simulink model "helicopter_sim"  (R2024b)
settings: Solver=ode4  StartTime=0.0  StopTime=30  FixedStep=ST  RelTol=1e-3
StopFcn:
  | % main rotor flapping restraint
  | if over_flap
  |     warning('MyModel:flapping', '<strong> main rotor blade flapping exceeded limits </strong>');
  | end
  | % tail rotor flapping restraint
  | if over_flap_tr
  |     warning('MyModel:flapping_tr', '<strong> tail rotor blade flapping exceeded limits </strong>');
  | end
  | % main rotor load limit
  | if load_mr
  |     warning('MyModel:load_mr', '<strong> main rotor load limit reached </strong>');
  | end
  | % main rotor power limit
  | if power_mr
  |     warning('MyModel:power_mr', '<strong> transmission maximum power rating reached </strong>');
  | end
  | % main rotor blade stall
  | if stall_mr
  |     warning('MyModel:blade_stall', '<strong> main rotor blade stall </strong>');
  | end
  | clear over_flap over_flap_tr load_mr power_mr stall_mr
values from neighbouring files (symbols this model uses):
  a_0 = [ 0 0 0 ]'*pi/180    [parameters.m]    (also in trim.m = [ flap_ss(1) flap_ss(2) flap_ss(3) ]')
  a_hs = 6    [parameters.m]
  a_vs = 6    [parameters.m]
  AKBETA = 0    [parameters.m]
  AKONE = 0    [parameters.m]
  AKONETR = tan(30*(pi/180))    [parameters.m]
  alpha_stall = 15    [parameters.m]
  AOP = 0    [parameters.m]
  AOPTR = 0    [parameters.m]
  AR_hs = 4.5    [parameters.m]
  AR_vs = 1.8    [parameters.m]
  ASLOPE = 6    [parameters.m]
  ASLOPETR = 6    [parameters.m]
  BLADES = 4    [parameters.m]
  BLADESTR = 3    [parameters.m]
  BLCG = 0    [parameters.m]
  BLHS = 0    [parameters.m]
  BLMR = 0    [parameters.m]
  BLRPF = 0    [parameters.m]
  BLTR = -1.8*Ft_m    (= -0.54864)    [parameters.m]
  BLVS = 0    [parameters.m]
  CD_f = [1.774 0.2043 7]    [parameters.m]
  CD_mr = [0.0107 -0.151 1.72]    [parameters.m]
  CD_tr = [ 0.0107 -0.151 1.72 ]    [parameters.m]
  chi_mr = 1    [parameters.m]
  chi_tr = 1    [parameters.m]
  CHORD = 2*Ft_m    (= 0.6096)    [parameters.m]
  CHORDTR = 1*Ft_m    (= 0.3048)    [parameters.m]
  CL_f = [-0.4279 10.33]    [parameters.m]
  CL_max_hs = 1.2    [parameters.m]
  CL_max_vs = 1.2    [parameters.m]
  CLL_f = [0.0696 6.336]    [parameters.m]
  CM_f = [-4.4961 49.522]    [parameters.m]
  CN_f = [0.0396 -21.699]    [parameters.m]
  CY_f = [-0.0359 -16.987]    [parameters.m]
  D = zeros(9,4)    [linearization.m]
  dyn_viscosity = 17.89e-6    (= 1.789e-05)    [parameters.m]
  e_hs = 0.8    [parameters.m]
  e_vs = 0.8    [parameters.m]
  EPSLN = 0.05    [parameters.m]
  euler0 = [ 0 0 0 ]'*pi/180    [parameters.m]    (also in trim.m = [ euler_trim(1)*abs(max_att) euler_trim(2)*abs(max_att) eule)
  fc = [  100*Kn_mps ... (first row only)    [parameters.m]
  GAMMA = 8.1    [parameters.m]
  GAMMATR = 4    [parameters.m]
  href = 0    [parameters.m]
  i_hs = -3*(pi/180)+a0_hs    (= -0.0523598775598)    [parameters.m]
  i_s = 0    [parameters.m]
  i_vs = 0*(pi/180)+a0_vs    (= -0.0872664625997)    [parameters.m]
  Jbeta = 1/3*m_blade*ROTOR^3*(1-EPSLN)^3    (= 3891.86391298)    [parameters.m]
  k_ind = 1    [parameters.m]
  k_ind_tr = 1    [parameters.m]
  kv_tr = 0.8    [parameters.m]
  Lambda_hs = 13*(pi/180)    (= 0.226892802759)    [parameters.m]
  Lambda_vs = 27*(pi/180)    (= 0.471238898038)    [parameters.m]
  lat_cyc_range = [ -15 15 ]    [parameters.m]
  latref = 39.24744998520548    (= 39.2474499852)    [parameters.m]
  lon_cyc_range = [ -15 15 ]    [parameters.m]
  lonref = 9.050782438199448    (= 9.0507824382)    [parameters.m]
  m = 20000*Lb_Kg    (= 9071.84)    [parameters.m]
  m_blade = 0.372*Slug_Kg/Ft_m    (= 17.8114564173)    [parameters.m]
  max_flap_mr = 20*pi/180    (= 0.349065850399)    [parameters.m]
  max_flap_tr = 20*pi/180    (= 0.349065850399)    [parameters.m]
  max_load = 3*m*9.81    (= 266984.2512)    [parameters.m]
  mode = 0    [linearization.m]    (also in parameters.m; trim.m)
  mr_coll_range = [   0 25 ]    [parameters.m]
  OMEGA = 206.9*(pi/30)    (= 21.6665173343)    [parameters.m]
  omega0 = [ 0 0 0 ]'    [parameters.m]
  OMEGATR = 954.93*(pi/30)    (= 100.000035756)    [parameters.m]
  pilot_trim = [ x(1); x(2); x(3); x(4) ]    [trim.m]
  rated_power = 4170*hp_W    (= 3109569)    [parameters.m]
  ROTOR = 30*Ft_m    (= 9.144)    [parameters.m]
  ROTORTR = 6.5*Ft_m    (= 1.9812)    [parameters.m]
  S_hs = 18*(Ft_m^2)    (= 1.67225472)    [parameters.m]
  S_vs = 33*(Ft_m^2)    (= 3.06580032)    [parameters.m]
  ST = 0.001    [parameters.m]
  STACG = 24.4*Ft_m    (= 7.43712)    [parameters.m]
  STAHS = 57.4*Ft_m    (= 17.49552)    [parameters.m]
  STAMR = 23.9*Ft_m    (= 7.28472)    [parameters.m]
  STARPF = 23.9*Ft_m    (= 7.28472)    [parameters.m]
  STATR = 61.4*Ft_m    (= 18.71472)    [parameters.m]
  STAVS = 59.4*Ft_m    (= 18.10512)    [parameters.m]
  THETT = -10*(pi/180)    (= -0.174532925199)    [parameters.m]
  THETTTR = -5*(pi/180)    (= -0.0872664625997)    [parameters.m]
  tr_coll_range = [   0 20 ]    [parameters.m]
  Ttrb = [ 1 0 0; 0 0 1; 0 -1 0]    [parameters.m]
  V0 = eul2rotm(euler0','XYZ')'*[ fc(1) fc(2) fc(3) ]'    [parameters.m]    (also in trim.m)
  wind_rate = [ 0 0 0 ]'    [parameters.m]
  wind_velocity_e = [ 0 0 0 ]'    [parameters.m]
  WLCG = 9.2*Ft_m    (= 2.80416)    [parameters.m]
  WLHS = 7.7*Ft_m    (= 2.34696)    [parameters.m]
  WLMR = 16.7*Ft_m    (= 5.09016)    [parameters.m]
  WLRPF = 12.2*Ft_m    (= 3.71856)    [parameters.m]
  WLTR = 15.2*Ft_m    (= 4.63296)    [parameters.m]
  WLVS = 12.2*Ft_m    (= 3.71856)    [parameters.m]
  Xe_0 = [ 16404 0 -1000 ]'*Ft_m    [parameters.m]
undefined symbols (not defined in the file or in its folder): Earth, rad, s, WGS84
libraries: simulink x4, aerolibanimutils x2, aerolibsim3d x2, sim3dlib x1, aerolibconvert2 x1, shared6dof x1, aerolibtransform2 x1, aerolibatmos2 x1
(part 2 of 3)

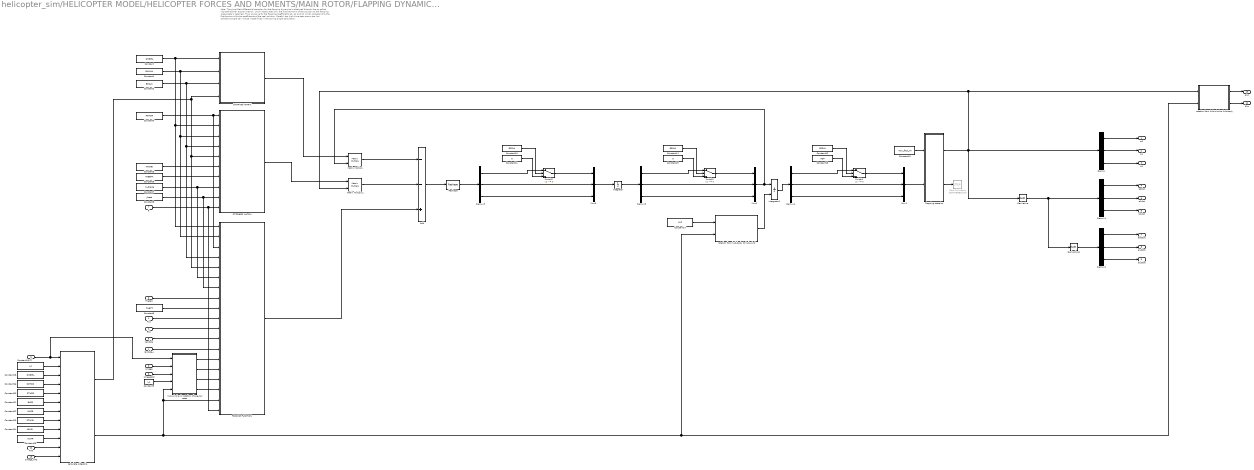
== system helicopter_sim/HELICOPTER MODEL/HELICOPTER FORCES AND MOMENTS/MAIN ROTOR/FLAPPING DYNAMICS (TIP-PATH-PLANE APPROX) ==
  note: Note:
      | The simplified differential equation for the flapping dynamics is obtained through the so called "tip-path-plane" approximation, which means that only the first harmonic of the solution to the flapping angle beta is retained. Thus we solve for the flapping coefficients a0, a1 and b1 which correspond to the first harmonic Fourier coefficients of the real solution.
      | Careful: too high time step size or too low collective angle can induce instabilities in the coning angle calculation.
  A1s : Inport
  B1s : Inport  Port=2
  Theta0 : Inport  Port=3
  lambda_i : Inport  Port=4
  lambda : Inport  Port=5
  chi : Inport  Port=6
  g : Inport  Port=7
  omegadot : Inport  Port=8
  omega : Inport  Port=9
  omega_TAS : Inport  Port=10
  TAS : Inport  Port=11
  Add : Sum  Inputs=--+
  Constant : Constant  Value=OMEGA
  Constant1 : Constant  Value=GAMMA
  Constant{2,10,12,14} (4 alike) : Constant  Value=EPSLN
  Constant11 : Constant  Value=0
  Constant13 : Constant  Value=AOP
  Constant15 : Constant  Value=0
  Constant16 : Constant  Value=max_flap_mr
  Constant17 : Constant  Value=a_0
  Constant18 : Constant  Value=OMEGA
  Constant19 : Constant  Value=i_s
  Constant20 : Constant  Value=STACG
  Constant21 : Constant  Value=BLCG
  Constant22 : Constant  Value=WLCG
  Constant23 : Constant  Value=STAMR
  Constant24 : Constant  Value=BLMR
  Constant25 : Constant  Value=WLMR
  Constant26 : Constant  Value=ROTOR
  Constant3 : Constant  Value=AKONE
  Constant4 : Constant  Value=ROTOR
  Constant5 : Constant  Value=THETT
  Constant6 : Constant  Value=AKBETA
  Constant7 : Constant  Value=m_blade
  Constant8 : Constant  Value=Jbeta
  Constant9 : Constant  Value=i_s
  DAMPING MATRIX : MATLAB Function  TreatAsAtomicUnit=on
  Demux{,1..5} (6 alike) : Demux  Outputs=3
  Derivative : Derivative
  Derivative1 : Derivative
  FORCING FUNCTION : MATLAB Function  TreatAsAtomicUnit=on
  Integrator : Integrator  InitialCondition=[0 0 0]'
  Integrator1 : Integrator  InitialConditionSource=external  InitialCondition=a_0
  Matrix Multiply : Product  Multiplication=Matrix(*)
  Matrix Multiply1 : Product  Multiplication=Matrix(*)
  Mux1 : Mux  Inputs=3
  Mux2 : Mux  Inputs=3
  Mux3 : Mux  Inputs=3
  Reshape : Reshape  OutputDimensionality=Column vector (2-D)
  STIFFNESS MATRIX : MATLAB Function  TreatAsAtomicUnit=on
  Stop Simulation : Stop  Commented=on
  Switch1 : Switch  Criteria=u2 ~= 0  SaturateOnIntegerOverflow=off  InputSameDT=off
  Switch2 : Switch  Criteria=u2 ~= 0  SaturateOnIntegerOverflow=off  InputSameDT=off
  Switch3 : Switch  Criteria=u2 ~= 0  SaturateOnIntegerOverflow=off  InputSameDT=off
  calculate sidesplip : MATLAB Function  TreatAsAtomicUnit=on
  flapping restraint : MATLAB Function  TreatAsAtomicUnit=on
  hub-wind axis rotation of angular rates : MATLAB Function  TreatAsAtomicUnit=on
  rotation from hub-body to hub-wind : MATLAB Function  TreatAsAtomicUnit=on
  rotation from hub-wind to hub-body : MATLAB Function  TreatAsAtomicUnit=on
  a0 : Outport
  a1 : Outport  Port=2
  b1 : Outport  Port=3
  a0dot : Outport  Port=4
  a1dot : Outport  Port=5
  b1dot : Outport  Port=6
  a0ddot : Outport  Port=7
  a1ddot : Outport  Port=8
  b1ddot : Outport  Port=9
  a1s : Outport  Port=10
  b1s : Outport  Port=11
  wires:
  Theta0/1 -> FORCING FUNCTION/8(Theta0)
  Constant2/1 -> DAMPING MATRIX/3(EPSLN), FORCING FUNCTION/4(EPSLN), STIFFNESS MATRIX/4(EPSLN)
  Constant1/1 -> DAMPING MATRIX/2(GAMMA), FORCING FUNCTION/2(GAMMA), STIFFNESS MATRIX/3(GAMMA)
  DAMPING MATRIX/1(D) -> Matrix Multiply/1
  Constant/1 -> FORCING FUNCTION/1(OMEGA), STIFFNESS MATRIX/2(OMEGA), DAMPING MATRIX/1(OMEGA)
  A1s/1 -> FORCING FUNCTION/10(A1s)
  FORCING FUNCTION/1(f) -> Add/3
  STIFFNESS MATRIX/1(K) -> Matrix Multiply1/1
  Constant5/1 -> FORCING FUNCTION/9(THETT)
  Matrix Multiply1/1 -> Add/2
  Demux/2 -> a1/1
  Matrix Multiply/1 -> Add/1
  Demux/1 -> a0/1
  Constant3/1 -> STIFFNESS MATRIX/6(AKONE)
  Demux/3 -> b1/1
  Add/1 -> Reshape/1
  B1s/1 -> FORCING FUNCTION/11(B1s)
  lambda/1 -> FORCING FUNCTION/12(lambda)
  Demux1/3 -> b1dot/1
  Demux1/1 -> a0dot/1
  Demux1/2 -> a1dot/1
  Demux2/2 -> a1ddot/1
  Demux2/1 -> a0ddot/1
  Demux2/3 -> b1ddot/1
  Constant6/1 -> STIFFNESS MATRIX/7(AKBETA)
  Constant7/1 -> STIFFNESS MATRIX/8(m_blade), FORCING FUNCTION/6(m_blade)
  Constant8/1 -> STIFFNESS MATRIX/9(Jbeta), FORCING FUNCTION/7(Jbeta)
  Constant4/1 -> STIFFNESS MATRIX/1(ROTOR), FORCING FUNCTION/3(ROTOR)
  rotation from hub-wind to hub-body/1(a1s) -> a1s/1
  rotation from hub-wind to hub-body/2(b1s) -> b1s/1
  omegadot/1 -> hub-wind axis rotation of angular rates/3(omegadot)
  hub-wind axis rotation of angular rates/1(pW) -> FORCING FUNCTION/14(pW)
  hub-wind axis rotation of angular rates/2(qW) -> FORCING FUNCTION/15(qW)
  hub-wind axis rotation of angular rates/3(pWdot) -> FORCING FUNCTION/16(pWdot)
  hub-wind axis rotation of angular rates/4(qWdot) -> FORCING FUNCTION/17(qWdot)
  omega/1 -> hub-wind axis rotation of angular rates/2(omega)
  Constant9/1 -> hub-wind axis rotation of angular rates/4(i_s)
  calculate sidesplip/1(Mu) -> DAMPING MATRIX/4(Mu), FORCING FUNCTION/5(Mu), STIFFNESS MATRIX/5(Mu)
  g/1 -> STIFFNESS MATRIX/10(g), FORCING FUNCTION/19(g)
  Constant15/1 -> Switch2/3
  Constant14/1 -> Switch2/2
  Demux5/3 -> Mux2/3
  Demux5/2 -> Mux2/2
  Demux5/1 -> Switch2/1
  Switch2/1 -> Mux2/1
  Integrator/1 -> Demux5/1  "adot"
  Mux2/1 -> Matrix Multiply/2, Integrator1/1
  Demux4/1 -> Switch1/1
  Constant13/1 -> Switch1/3
  Constant12/1 -> Switch1/2
  Integrator1/1 -> Demux4/1  "a"
  flapping restraint/1(a) -> Derivative/1, Demux/1, Matrix Multiply1/2, rotation from hub-wind to hub-body/1(a)
  Switch3/1 -> Mux3/1
  Demux3/2 -> Mux3/2
  Demux3/3 -> Mux3/3
  Constant11/1 -> Switch3/3
  Demux3/1 -> Switch3/1
  Constant10/1 -> Switch3/2
  Reshape/1 -> Demux3/1  "addot"
  Mux3/1 -> Integrator/1
  Derivative/1 -> Demux1/1, Derivative1/1
  Derivative1/1 -> Demux2/1
  lambda_i/1 -> FORCING FUNCTION/13(lambda_i)
  Switch1/1 -> Mux1/1
  Demux4/2 -> Mux1/2
  Demux4/3 -> Mux1/3
  Mux1/1 -> flapping restraint/2("a ")
  Constant16/1 -> flapping restraint/1(max_flap)
  flapping restraint/2(stop) -> Stop Simulation/1
  rotation from hub-body to hub-wind/1(a_w) -> Integrator1/2
  Constant17/1 -> rotation from hub-body to hub-wind/1(a_b)
  chi/1 -> hub-wind axis rotation of angular rates/1(chi), calculate sidesplip/1(chi)
  Constant19/1 -> calculate sidesplip/2(i_s)
  Constant20/1 -> calculate sidesplip/5(STACG)
  Constant21/1 -> calculate sidesplip/6(BLCG)
  Constant22/1 -> calculate sidesplip/7(WLCG)
  Constant23/1 -> calculate sidesplip/8(STAH)
  Constant24/1 -> calculate sidesplip/9(BLH)
  Constant25/1 -> calculate sidesplip/10(WLH)
  TAS/1 -> calculate sidesplip/11(TAS)
  Constant18/1 -> calculate sidesplip/3(OMEGA)
  Constant26/1 -> calculate sidesplip/4(ROTOR)
  omega_TAS/1 -> calculate sidesplip/12(omega_TAS)
  calculate sidesplip/2(beta_w) -> FORCING FUNCTION/18(beta_w), hub-wind axis rotation of angular rates/5(beta_w), rotation from hub-body to hub-wind/2(beta_w), rotation from hub-wind to hub-body/2(beta_w)

== system helicopter_sim/HELICOPTER MODEL/HELICOPTER FORCES AND MOMENTS/MAIN ROTOR/Stop simulation if retreating blade stalls  ==
  alpha_loc : Inport
  Compare To Constant : simulink/Logic and Bit Operations/Compare To Constant  relop=>  const=alpha_stall  OutDataTypeStr=boolean
  Display : Display
  MATLAB Function : MATLAB Function  TreatAsAtomicUnit=on
  MATLAB Function1 : MATLAB Function  TreatAsAtomicUnit=on
  Stop Simulation : Stop  Commented=on
  wires:
  Compare To Constant/1 -> MATLAB Function/1(u), Stop Simulation/1
  alpha_loc/1 -> MATLAB Function1/1(alpha_loc)
  MATLAB Function1/1(alpha_max) -> Display/1, Compare To Constant/1

== system helicopter_sim/HELICOPTER MODEL/HELICOPTER FORCES AND MOMENTS/MAIN ROTOR/Stop simulation if main rotor hub load limit is exceeded ==
  T : Inport
  Compare To Constant : simulink/Logic and Bit Operations/Compare To Constant  relop=>  const=max_load  OutDataTypeStr=boolean
  MATLAB Function : MATLAB Function  TreatAsAtomicUnit=on
  Scope : Scope
  Stop Simulation : Stop  Commented=on
  wires:
  Compare To Constant/1 -> MATLAB Function/1(u), Stop Simulation/1
  T/1 -> Scope/1, Compare To Constant/1

== system helicopter_sim/HELICOPTER MODEL/HELICOPTER FORCES AND MOMENTS/MAIN ROTOR/Stop simulation if maximum transmission power rating is exceeded ==
  Q : Inport
  Compare To Constant : simulink/Logic and Bit Operations/Compare To Constant  relop=>  const=rated_power  OutDataTypeStr=boolean
  Constant : Constant  Value=OMEGA
  MATLAB Function : MATLAB Function  TreatAsAtomicUnit=on
  Product : Product
  Scope : Scope
  Stop Simulation : Stop  Commented=on
  wires:
  Compare To Constant/1 -> MATLAB Function/1(u), Stop Simulation/1
  Q/1 -> Product/1
  Constant/1 -> Product/2
  Product/1 -> Compare To Constant/1, Scope/1

== matlab function helicopter_sim/HELICOPTER MODEL/HELICOPTER FORCES AND MOMENTS/STABILIZERS /VERTICAL STABILIZER AERODYNAMIC FORCES AND MOMENTS ==
  data: lambda_i_tr input; TAS input; omega_TAS input; rho input; STAVS input; F_vs output; BLVS input; WLVS input; STACG input; BLCG input; WLCG input; OMEGATR input; ROTORTR input; i_vs input; S_vs input; AR_vs input; CL_max input; e_vs input; a_vs input; Lambda_vs input; kv_tr input; M_vs output
function [F_vs,M_vs] = fcn(lambda_i_tr,TAS,omega_TAS,rho,STAVS,BLVS,WLVS,STACG,BLCG,WLCG,OMEGATR,ROTORTR,...
                           i_vs,S_vs,AR_vs,CL_max,e_vs,a_vs,Lambda_vs,kv_tr)

%% preliminary calculations
% tail rotor downwash on horizontal stabilizer:
% simply the value of induced velocity at the rotor disk times a correction factor accounting for how much of the stabilizer is inside the wake and on which side it is
% reminder: induced velocity ratio is positive when going from left to right through the tail rotor
if (lambda_i_tr*kv_tr)<0 % consider induced velocity only if the stabilizer is inside the wake
    v_i = -lambda_i_tr*OMEGATR*ROTORTR*abs(kv_tr);
else
    v_i = 0;
end
% velocity in body axis:
lever_arm = [STACG-STAVS BLVS-BLCG WLCG-WLVS]'; % vector from cg to stabilizer
TAS_VS = (TAS + cross(omega_TAS,lever_arm)); % apparent wind speed at stabilizer
u_vs = TAS_VS(1);
v_vs = TAS_VS(2)+v_i;
w_vs = TAS_VS(3);
V_vs = sqrt(u_vs^2+v_vs^2+w_vs^2);
q = 0.5*rho*V_vs^2;
% angle of attack:
alpha_vs = atan2(v_vs,u_vs)+i_vs;
if V_vs == 0
    beta_vs = 0;
else
    beta_vs = asin(w_vs/V_vs);
end

%% aerodynamic coefficients:
a_vs3D = a_vs/(1+a_vs/(pi*AR_vs*e_vs))*cos(beta_vs+Lambda_vs)^2;% lift curve slope (lifting line theory corrected for sideslip and sweep)
if (CL_max/a_vs3D)<pi/4
    alpha_stall = CL_max/a_vs3D;
else 
    alpha_stall = pi/4;
    CL_max = a_vs3D*pi/4;
end
alpha_1 = 1.2*alpha_stall;
alpha_i = NaN;
if 0<=alpha_vs && alpha_vs<pi/2
    alpha_i = alpha_vs;
elseif -pi/2<=alpha_vs && alpha_vs<0
    alpha_i = -alpha_vs;
elseif pi/2<=alpha_vs && alpha_vs<pi
    alpha_i = pi-alpha_vs;
elseif -pi<=alpha_vs && alpha_vs<-pi/2
    alpha_i = pi+alpha_vs;
end
% lift:
CL_0 = NaN;
if 0<=alpha_i && alpha_i<alpha_stall
    CL_0 = a_vs3D*alpha_i;
elseif alpha_stall<=alpha_i && alpha_i<alpha_1
    CL_0 = CL_max-a_vs3D*(alpha_i-alpha_stall);
elseif alpha_1<=alpha_i && alpha_i<=pi/2
    CL_0 = 0.8*CL_max*(1-((alpha_i-alpha_1)/(pi/2-alpha_1))^2);
end
CL_vs = NaN;
if 0<=alpha_vs && alpha_vs<pi/2
    CL_vs = CL_0;
elseif -pi/2<=alpha_vs && alpha_vs<0
    CL_vs = -CL_0;
elseif pi/2<=alpha_vs && alpha_vs<pi
    CL_vs = -0.8*CL_0;
elseif -pi<=alpha_vs && alpha_vs<-pi/2
    CL_vs = 0.8*CL_0;
end
% drag:
CD_p = NaN;
if 0<=alpha_i && alpha_i<=0.35
    CD_p = 0.009+0.11*alpha_i^2;
elseif 0.35<alpha_i && alpha_i<pi/2
    CD_p = -0.1254+0.9415*alpha_i+0.977525*sin(alpha_i)^2;
end
CD_vs = CD_p+CL_vs^2/(e_vs*pi*AR_vs);

%% forces calculation in body axis:
X_vs = q*S_vs*(-CD_vs*cos(alpha_vs)*cos(beta_vs)+CL_vs*sin(alpha_vs));
Y_vs = q*S_vs*(-CL_vs*cos(alpha_vs)-CD_vs*sin(alpha_vs)*cos(beta_vs));
Z_vs = q*S_vs*(-CD_vs*sin(beta_vs));
F_vs = [ X_vs, Y_vs, Z_vs ]';

%% moments around cg:
M_vs = cross(lever_arm,F_vs);

== matlab function helicopter_sim/HELICOPTER MODEL/HELICOPTER FORCES AND MOMENTS/CONTROL MIXER/DIMENSIONALIZATION ==
  data: deltaA input; deltaB input; deltaC input; deltaP input; lat_cyc output; lon_cyc output; mr_coll output; tr_coll output; lat_cyc_range input; lon_cyc_range input; mr_coll_range input; tr_coll_range input
function [lat_cyc,lon_cyc,mr_coll,tr_coll] = fcn(deltaA,deltaB,deltaC,deltaP,lat_cyc_range,lon_cyc_range,mr_coll_range,tr_coll_range)

lat_cyc = (deltaA*0.5*(lat_cyc_range(2)-lat_cyc_range(1))+0.5*(lat_cyc_range(2)+lat_cyc_range(1)))*pi/180;
lon_cyc = (deltaB*0.5*(lon_cyc_range(2)-lon_cyc_range(1))+0.5*(lon_cyc_range(2)+lon_cyc_range(1)))*pi/180;
mr_coll = (deltaC*0.5*(mr_coll_range(2)-mr_coll_range(1))+0.5*(mr_coll_range(2)+mr_coll_range(1)))*pi/180;
tr_coll = (deltaP*0.5*(tr_coll_range(2)-tr_coll_range(1))+0.5*(tr_coll_range(2)+tr_coll_range(1)))*pi/180;

== matlab function helicopter_sim/HELICOPTER MODEL/HELICOPTER FORCES AND MOMENTS/STABILIZERS /HORIZONTAL STABILIZER AERODYNAMIC FORCES AND MOMENTS ==
  data: lambda_i input; TAS input; omega_TAS input; F_hs output; rho input; STAHS input; BLHS input; WLHS input; STACG input; BLCG input; WLCG input; OMEGA input; ROTOR input; i_hs input; S_hs input; AR_hs input; CL_max input; e_hs input; a_hs input; M_hs output; Lambda_hs input
function [F_hs,M_hs] = fcn(lambda_i,TAS,omega_TAS,rho,STAHS,BLHS,WLHS,STACG,BLCG,WLCG,OMEGA,ROTOR,...
                           i_hs,S_hs,AR_hs,CL_max,e_hs,a_hs,Lambda_hs)

%% preliminary calculations
% main rotor downwash on horizontal stabilizer:
% simply double the value of induced velocity at the rotor disk (the stabilizer is considered to be placed in the completely developed wake)
% reminder: induced velocity ratio is positive when going up through the main rotor
w_ihs = 2*(lambda_i)*OMEGA*ROTOR;
% velocity in body axis:
lever_arm = [STACG-STAHS BLHS-BLCG WLCG-WLHS]'; % vector from cg to stabilizer
TAS_HS = (TAS + cross(omega_TAS,lever_arm)); % apparent wind speed at stabilizer
u_hs = TAS_HS(1);
v_hs = TAS_HS(2);
w_hs = TAS_HS(3)+w_ihs;
V_hs = sqrt(u_hs^2+v_hs^2+w_hs^2);
q = 0.5*rho*V_hs^2;
% angle of attack:
alpha_hs = atan2(w_hs,u_hs)+i_hs;
if V_hs == 0
    beta_hs = 0;
else
    beta_hs = asin(v_hs/V_hs);
end

%% aerodynamic coefficients:
a_hs3D = a_hs/(1+a_hs/(pi*AR_hs*e_hs))*cos(beta_hs+Lambda_hs)^2;% lift curve slope (lifting line theory corrected for sideslip)
if (CL_max/a_hs3D)<pi/4
    alpha_stall = CL_max/a_hs3D;
else 
    alpha_stall = pi/4;
    CL_max = a_hs3D*pi/4;
end
alpha_1 = 1.2*alpha_stall;
alpha_i = NaN;
if 0<=alpha_hs && alpha_hs<pi/2
    alpha_i = alpha_hs;
elseif -pi/2<=alpha_hs && alpha_hs<0
    alpha_i = -alpha_hs;
elseif pi/2<=alpha_hs && alpha_hs<pi
    alpha_i = pi-alpha_hs;
elseif -pi<=alpha_hs && alpha_hs<-pi/2
    alpha_i = pi+alpha_hs;
end
% lift:
CL_0 = NaN;
if 0<=alpha_i && alpha_i<alpha_stall
    CL_0 = a_hs3D*alpha_i;
elseif alpha_stall<=alpha_i && alpha_i<alpha_1
    CL_0 = CL_max-a_hs3D*(alpha_i-alpha_stall);
elseif alpha_1<=alpha_i && alpha_i<=pi/2
    CL_0 = 0.8*CL_max*(1-((alpha_i-alpha_1)/(pi/2-alpha_1))^2);
end
CL_hs = NaN;
if 0<=alpha_hs && alpha_hs<pi/2
    CL_hs = CL_0;
elseif -pi/2<=alpha_hs && alpha_hs<0
    CL_hs = -CL_0;
elseif pi/2<=alpha_hs && alpha_hs<pi
    CL_hs = -0.8*CL_0;
elseif -pi<=alpha_hs && alpha_hs<-pi/2
    CL_hs = 0.8*CL_0;
end
% drag:
CD_p = NaN;
if 0<=alpha_i && alpha_i<=0.35
    CD_p = 0.009+0.11*alpha_i^2;
elseif 0.35<alpha_i && alpha_i<pi/2
    CD_p = -0.1254+0.9415*alpha_i+0.977525*sin(alpha_i)^2;
end
CD_hs = CD_p+CL_hs^2/(e_hs*pi*AR_hs);

%% forces calculation in body axis:
X_hs = q*S_hs*(-CD_hs*cos(beta_hs)*cos(alpha_hs)+CL_hs*sin(alpha_hs));
Y_hs = q*S_hs*(-CD_hs*sin(beta_hs));
Z_hs = q*S_hs*(-CL_hs*cos(alpha_hs)-CD_hs*cos(beta_hs)*sin(alpha_hs));
F_hs = [ X_hs, Y_hs, Z_hs ]';

%% moments around cg:
M_hs = cross(lever_arm,F_hs);

== matlab function helicopter_sim/HELICOPTER MODEL/HELICOPTER FORCES AND MOMENTS/TAIL ROTOR /AERODYNAMIC AND INERTIAL FORCES AND MOMENTS ==
  data: chi input; AOP input; Ttrb input; m_blade input; Jbeta input; GAMMA input; EPSLN input; AKBETA input; g input; BLADES input; Mrotor output; ASLOPE input; AKONE input; CHORD input; CD input; ROTOR input; Theta0 input; THETT input; dyn_viscosity input; k_ind input; STACG input; BLCG input; WLCG input; STAH input; BLH input; WLH input; rho input; TAS input; omega_TAS input; Frotor output; omega input; OMEGA input; lambda_i output; max_flap input; T output
function [Mrotor,Frotor,lambda_i,T]  = fcn(chi,AOP,Ttrb,m_blade,Jbeta,GAMMA,EPSLN,AKBETA,g,BLADES,ASLOPE,AKONE,CHORD,CD,ROTOR,...
                                         Theta0,THETT,dyn_viscosity,k_ind,...
                                         STACG,BLCG,WLCG,STAH,BLH,WLH,rho,TAS,omega_TAS,omega,OMEGA,max_flap)

%% preliminary calculations
% assumptions and simplifications:
% teetering rotor, flapping dynamics neglected due to high angular speed,
% coning equal to fixed pre-cone angle,
% no cyclic pitch, effect of downwash of main rotor not considered
A1c = 0; B1c = 0; a0 = AOP;
a0dot = 0; a0ddot = 0;
a1dot = 0; a1ddot = 0;
b1dot = 0; b1ddot = 0;
A = pi*ROTOR^2; % area of rotor disc 
sigma = BLADES*CHORD/(pi*ROTOR); % solidity of rotor 
lever_arm_H = [STACG-STAH BLH-BLCG WLCG-WLH]'; % vector from cg to rotor hub
TAS_H = (TAS + cross(omega_TAS,lever_arm_H)); % wind speed at rotor
% rotation of airspeed from body to hub-body frame:
TAS_H = Ttrb*TAS_H(:);
uH = TAS_H(1);
vH = TAS_H(2);
wH = TAS_H(3);
beta_w = atan2(vH,uH); % sideslip angle 
Mu = sqrt(uH^2+vH^2)/(OMEGA*ROTOR); % advance ratio
% rotation of body angular rates from body to hub-body frame:
omegaH = Ttrb*omega(:);
pH = omegaH(1); % roll rate in hub axis
qH = omegaH(2); % pitch rate in hub axis
% rotation of body angular rates from hub-body to hub-wind frame:
pW = pH*cos(beta_w)+qH*sin(beta_w);
qW = -pH*sin(beta_w)+qH*cos(beta_w);
% rotation of feathering angles from hub-body to hub-wind frame:
Mbeta = g*1/2*m_blade*ROTOR^2*(1-EPSLN)^2; % weight moment of the blade around flap hinge (small flapping angle beta and level attitude) 
                                           % (distance from blade c.g. to flap hinge)*(blade weight) [N*m]
                                           % small contribution to the coning angle, can be neglected


%% iteration between inflow and flapping calculations
% starting guess:
lambda = -0.1; lambda_i = -0.1; T = 0; delta = 0;
a1 = 0; b1 = 0; 

iter = true;
it = 0; %counter
tol = 0.001; %tolerance as fraction of control variable
flag = false; 
while iter == true

    %% steady inherent flapping calculation
    a10 = a1; b10 = b1; % store previous step 
    Delta = 1-Mu^4/4+AKONE^2*(1+Mu^2/2)*(1+3/2*Mu^2);
    f1 = 4/3*Mu*a0-16/(GAMMA*OMEGA)*pH-qH/OMEGA;
    f2 = 8/3*AKONE*Mu*a0+16*qH/(GAMMA*OMEGA)-Mu*(8/3*Theta0+2*THETT+2*lambda-pH/OMEGA);
    a1 = 1/Delta*(AKONE*(1+3/2*Mu^2)*f1-(1+Mu^2/2)*f2);
    b1 = 1/Delta*((1-Mu^2/2)*f1+AKONE*(1+Mu^2/2)*f2);

    % iteration control:
    it = it +1; % counter
    % ending criterion:
    diff = [abs(a1-a10) abs(b1-b10)]; 
    if it>5
        if diff(1)<=abs(tol*a1) && diff(2)<=abs(tol*b1)
            iter = false;

            % set limits to flapping angles:
            beta_max = a0 + sqrt(a1^2+b1^2);
            beta_min = a0 - sqrt(a1^2+b1^2);
            if abs(beta_max)>max_flap ||  abs(beta_min)>max_flap
                
                k = sqrt((max_flap-abs(a0))^2)/sqrt(a1^2+b1^2); %scaling factor (coning unaltered)
                a1 = k*a1; b1 = k*b1;
                flag = true;
            end

        elseif it>=1000
            iter = false;
            a1 = 0; b1 = 0;
            fprintf(['<strong> WARNING: calculation of tail rotor flapping angles does not converge  </strong> \n ' ...
                     ' reverting to calculation without considering flapping'])
        end
    end
    

    %% thrust and inflow calculation
    
    lambda = fzero(@(x) x-wH/(OMEGA*ROTOR)+0.5*(0.5*BLADES*rho*ASLOPE*CHORD*ROTOR*(OMEGA*ROTOR)^2*(1/2*(1-EPSLN^2)*x+Theta0*(1/3+Mu^2/2*(1-EPSLN))+THETT*(1/4+Mu^2/4*(1-EPSLN^2))+...
                        -Mu/2*(1-EPSLN^2)*(B1c-AKONE*b1)-a0*(1/3+Mu^2/2*(1-EPSLN))*AKONE+a1*(Mu/2*EPSLN*(1-EPSLN))-a0dot/OMEGA*(1/3-EPSLN/2)+b1dot/OMEGA*(Mu/4*(1-EPSLN)^2)+...
                        +Mu/4*(1-EPSLN^2)*pW/OMEGA)-BLADES*Mbeta/g*a0ddot)/(rho*A*(OMEGA*ROTOR)^2)/sqrt(Mu^2+x^2), -0.1);
    vi = wH-lambda*OMEGA*ROTOR;
    lambda_i = -vi/OMEGA/ROTOR;
    T =  0.5*BLADES*rho*ASLOPE*CHORD*ROTOR*(OMEGA*ROTOR)^2*(1/2*(1-EPSLN^2)*lambda+Theta0*(1/3+Mu^2/2*(1-EPSLN))+THETT*(1/4+Mu^2/4*(1-EPSLN^2))+...
         -Mu/2*(1-EPSLN^2)*(B1c-AKONE*b1)-a0*(1/3+Mu^2/2*(1-EPSLN))*AKONE+a1*(Mu/2*EPSLN*(1-EPSLN))-a0dot/OMEGA*(1/3-EPSLN/2)+b1dot/OMEGA*(Mu/4*(1-EPSLN)^2)+...
         +Mu/4*(1-EPSLN^2)*pW/OMEGA)-BLADES*Mbeta/g*a0ddot;
    CT = T/(rho*A*(OMEGA*ROTOR)^2);
    V = sqrt(vi^2+(OMEGA*ROTOR)^2);
    Re = rho*CHORD*V/dyn_viscosity; % Reynolds number based on tip speed and rotor chord
    alpha_mean = 6*CT/ASLOPE/sigma;
    delta = CD(1)+CD(2)*alpha_mean+CD(3)*alpha_mean^2;

end

if flag
    over_flap_tr = true;
    assignin('base', 'over_flap_tr', over_flap_tr);
else
    over_flap_tr = false;
    assignin('base', 'over_flap_tr', over_flap_tr);
end

%% forces and moments in the hub-wind frame

H_w = BLADES/2*rho*ASLOPE*CHORD*ROTOR*(OMEGA*ROTOR)^2*(delta*Mu/(2*ASLOPE)*(1-EPSLN^2)-1/4*(Theta0-AKONE*a0)*(2*lambda*Mu*(1-EPSLN)+ ...
      -Mu*(1-EPSLN)^2*a0dot/OMEGA-(EPSLN-2/3)*(b1dot/OMEGA-a1)-2/3*a1+2/3*pW/OMEGA)-THETT/4*(Mu*lambda*(1-EPSLN^2)+a0dot/OMEGA*Mu*(EPSLN-2/3)+...
      -2*(EPSLN/3-1/4)*(b1dot/OMEGA-a1)-a1/2+1/2*pW/OMEGA)+1/4*(A1c-AKONE*a1)*(-b1*Mu/4*(1-EPSLN^2)+1/4*Mu*(1-EPSLN)^2*(a1dot/OMEGA+b1)+2/3*a0+...
      +Mu/4*(1-EPSLN^2)*qW/OMEGA)+1/4*(B1c-AKONE*b1)*(3/4*Mu*(1-EPSLN)^2*(b1dot/OMEGA-a1)+(1-EPSLN^2)*(lambda-a1*Mu/4)+(EPSLN-2/3)*a0dot/OMEGA+...
      +3*Mu/4*(1-EPSLN^2)*pW/OMEGA)+1/4*(EPSLN*(1-EPSLN)*(b1dot/OMEGA-a1)*4*lambda-(1-EPSLN^2)*(2*lambda*(b1dot/OMEGA-a1)-a1*lambda)+...
      -(2/3-EPSLN)*(a1*a0dot/OMEGA+a0*(a1dot/OMEGA+b1))-2*a0/3*qW/OMEGA-(2*(1-EPSLN^2)*lambda-4*(1/3-EPSLN/2)*a0dot/OMEGA)*pW/OMEGA+...
      +4*a0dot/OMEGA*(b1dot/OMEGA-a1)*(1/3-EPSLN+EPSLN^2))+Mu/4*(EPSLN*(1-EPSLN)*(a1*(b1dot/OMEGA-a1)+b1*(a1dot/OMEGA+b1))+...
      +1/4*(1-EPSLN)^2*(b1*(a1dot/OMEGA+b1)+a1*(b1dot/OMEGA-a1))-1/2*(1-EPSLN^2)*(a1*(b1dot/OMEGA-a1)+b1*(a1dot/OMEGA+b1)-2*a0^2-b1^2/2-3/2*a1^2)+...
      -a1/4*(1-EPSLN^2)*pW/OMEGA-b1/4*(1-EPSLN^2)*qW/OMEGA));

Y_w = BLADES/2*rho*ASLOPE*CHORD*ROTOR*(OMEGA*ROTOR)^2*(-1/4*(Theta0-AKONE*a0)*(((EPSLN-2/3)*(a1dot/OMEGA+b1)-2/3*b1)+3*a0*(1-EPSLN^2)*Mu+ ...
      -2*b1*(1-EPSLN)*Mu^2-2/3*qW/OMEGA)-THETT/4*(((2/3*EPSLN-1/2)*(a1dot/OMEGA+b1)-b1/2)+2*a0*Mu-b1*(1-EPSLN^2)*Mu^2+ ...
      -1/2*qW/OMEGA)-1/4*(A1c-AKONE*a1)*(((EPSLN-2/3)*a0dot/OMEGA+lambda*(1-EPSLN^2))+Mu*(5/4*a1*(1-EPSLN^2)+1/4*(1-EPSLN)^2*(b1dot/OMEGA-a1))+...
      +Mu/4*(1-EPSLN^2)*pW/OMEGA)-1/4*(B1c-AKONE*b1)*(-2/3*a0+Mu*(7/4*b1*(1-EPSLN^2)+1/4*(1-EPSLN)^2*(a1dot/OMEGA+b1)+...
      +1/4*qW/OMEGA)-Mu^2*(2*a0*(1-EPSLN)))-1/4*(4*(1/3-EPSLN+EPSLN^2)*a0dot/OMEGA*(a1dot/OMEGA+b1)-2*lambda*(1-EPSLN)^2*(a1dot/OMEGA+b1)+...
      +2/3*a0*pW/OMEGA+2*a0*(1/3-EPSLN/2)*(b1dot/OMEGA-a1)-2*b1*(lambda/2*(1-EPSLN^2)-a0dot/OMEGA*(1/3-EPSLN/2))+(4*(1/3-EPSLN/2)*a0dot/OMEGA+...
      -2*(1-EPSLN^2)*lambda)*qW/OMEGA)-Mu/4*(6*a0*lambda*(1-EPSLN)-a1*b1/2*(1-EPSLN^2)-3*(1-EPSLN)^2*a0*a0dot/OMEGA-7/4*(1-EPSLN)^2*a1*(a1dot/OMEGA+b1)+...
      -5/4*b1*(1-EPSLN^2)*pW/OMEGA-7/4*a1*(1-EPSLN^2)*qW/OMEGA-5/4*(1-EPSLN)^2*b1*(b1dot/OMEGA-a1))-Mu^2*(a0*a1*(1-EPSLN)));

M_w = BLADES/2*(AKBETA*a1-EPSLN*ROTOR*Mbeta/g*(a1ddot+2*b1dot*OMEGA-a1*OMEGA^2))-BLADES/2*Jbeta*OMEGA^2*GAMMA*EPSLN*(-(1/6+Mu^2/8*(1-EPSLN))*(A1c-AKONE*a1)+...
      -Mu/4*(1-EPSLN^2)*a0+Mu^2/8*(1-EPSLN)*b1+(1/6-EPSLN/4)*(a1dot/OMEGA+b1)+1/6*qW/OMEGA);

L_w = BLADES/2*(AKBETA*b1-EPSLN*ROTOR*Mbeta/g*(b1ddot-2*a1dot*OMEGA-b1*OMEGA^2))-BLADES/2*Jbeta*OMEGA^2*GAMMA*EPSLN*(Mu/2*(1-EPSLN^2)*(Theta0-AKONE*a0)+...
      -(1/6+3/8*Mu^2*(1-EPSLN))*(B1c-AKONE*b1)+Mu/3*THETT+Mu/2*(1-EPSLN)*lambda+Mu^2/8*(1-EPSLN)*a1-Mu/4*(1-EPSLN)^2*a0dot/OMEGA+(1/6-EPSLN/4)*(b1dot/OMEGA-a1)+1/6*pW/OMEGA);

Q = k_ind*BLADES/2*rho*ASLOPE*CHORD*ROTOR^2*(OMEGA*ROTOR)^2*(delta/k_ind/(4*ASLOPE)*(1+(1-EPSLN^2)*Mu^2)-(Theta0-AKONE*a0)*(lambda/3+(EPSLN/3-1/4)*a0dot/OMEGA+...
    +Mu/6*b1dot/OMEGA-Mu*EPSLN/4*(b1dot/OMEGA-a1)+Mu/6*pW/OMEGA)+(A1c-AKONE*a1)*((1/8-EPSLN/6)*(a1dot/OMEGA+b1)-Mu/6*a0+b1/16*(1-EPSLN^2)*Mu^2+1/8*qW/OMEGA)+...
    +(B1c-AKONE*b1)*((1/8-EPSLN/6)*(b1dot/OMEGA-a1)+(EPSLN/4-1/6)*Mu*a0dot/OMEGA+1/2*(1-EPSLN^2)*(Mu*lambda/2+a1/8*Mu^2)+1/8*pW/OMEGA)-THETT*(lambda/4+...
    +(EPSLN/4-1/5)*a0dot/OMEGA+Mu/8*b1dot/OMEGA-EPSLN*Mu/6*(b1dot/OMEGA-a1))-1/2*(1-EPSLN^2)*(lambda^2+lambda*Mu*a1+2*lambda*EPSLN*a0dot/OMEGA+...
    +Mu*EPSLN*(a1*a0dot/OMEGA+a0*(a1dot/OMEGA+b1))+Mu^2*(a0^2/2+3/8*a1^2+1/8*b1^2))+Mu/3*(a1*a0dot/OMEGA+a0*(a1dot/OMEGA+b1))+2/3*lambda*a0dot/OMEGA+...
    -(-Mu/3*a0+(1/4-EPSLN/3)*(a1dot/OMEGA+b1))*qW/OMEGA-(1/4-EPSLN/3)*(b1/OMEGA-a1)*pW/OMEGA-1/8*(qW/OMEGA)^2-1/8*(pW/OMEGA)^2-(1/4-2/3*EPSLN+EPSLN^2/2)*((a0dot/OMEGA)^2+...
    +1/2*((a1dot/OMEGA+b1)^2+(b1dot/OMEGA-a1)^2)));


%% back rotation from hub_wind frame to hub-frame

H_H = H_w*cos(beta_w)+Y_w*sin(beta_w);
Y_H = -H_w*sin(beta_w)+Y_w*cos(beta_w);
L_H = L_w*cos(beta_w)-M_w*sin(beta_w);
M_H = L_w*sin(beta_w)+M_w*cos(beta_w);

%% back rotation from hub-frame to body-frame

Frotor = Ttrb'*[ -H_H Y_H -T ]';
Mrotor = Ttrb'*[ L_H M_H Q ]' + cross(lever_arm_H,Frotor);

== matlab function helicopter_sim/HELICOPTER MODEL/HELICOPTER FORCES AND MOMENTS/CONTROL MIXER/CYCLIC MIXING MATRIX ==
  data: mixing_matrix output; ROTOR input; EPSLN input; m_blade input; AKBETA input; Jbeta input; OMEGA input; AKONE input; GAMMA input
function mixing_matrix = fcn(ROTOR,EPSLN,m_blade,AKBETA,Jbeta,OMEGA,AKONE,GAMMA)

% preliminary calculations:
g = 9.81; % gravity acc. considered constant for the porpouse of control mixing law [m/s^2]
Mbeta = g*1/2*m_blade*ROTOR^2*(1-EPSLN)^2; % weight moment of the blade around flap hinge (small flapping angle beta and level attitude) 
                                           % (distance from blade c.g. to flap hinge)*(blade weight) [N*m]
                                           % small contribution to the coning angle, can be neglected
P2 = 1 + AKBETA/(Jbeta*OMEGA^2) + EPSLN*ROTOR*Mbeta/(Jbeta*g) + GAMMA*AKONE/8*(1-4/3*EPSLN); % squared ratio of flapping frequency and rotor angular speed

A1s_deltaA = (1-8/3*EPSLN+2*EPSLN^2)/(1-4/3*EPSLN);
B1s_deltaA = (8*(P2-1))/(GAMMA*(1-4/3*EPSLN));
A1s_deltaL = (8*(P2-1))/(GAMMA*(1-4/3*EPSLN));
B1s_deltaL = -(1-8/3*EPSLN+2*EPSLN^2)/(1-4/3*EPSLN);

mixing_matrix = [ A1s_deltaA A1s_deltaL ;
                  B1s_deltaA B1s_deltaL ];

% mixing_matrix = [1  0;
%                  0 -1];

== matlab function helicopter_sim/HELICOPTER MODEL/HELICOPTER FORCES AND MOMENTS/MAIN ROTOR/Stop simulation if maximum transmission power rating is exceeded/MATLAB Function ==
  data: u input
function fcn(u)

if u
    power_mr = true;
    assignin('base', 'power_mr', power_mr);
else
    power_mr = false;
    assignin('base', 'power_mr', power_mr);
end

== matlab function helicopter_sim/GCS gamepad/indexing for manual control ==
  data: u input; y output
function y = fcn(u)

% index for manual control:
y = [ u(2) u(3) u(1) -u(4) ]';

== matlab function helicopter_sim/HELICOPTER MODEL/HELICOPTER FORCES AND MOMENTS/MAIN ROTOR/Stop simulation if main rotor hub load limit is exceeded/MATLAB Function ==
  data: u input
function fcn(u)

if u
    load_mr = true;
    assignin('base', 'load_mr', load_mr);
else
    load_mr = false;
    assignin('base', 'load_mr', load_mr);
end

== matlab function helicopter_sim/HELICOPTER MODEL/Stop Simulation at Ground Level/MATLAB Function ==
  data: u input
function fcn(u)

if u==true
    fprintf('GROUND LIMIT REACHED: SIMULATION STOPPED')
end

== matlab function helicopter_sim/GCS gamepad/ exponential scaling  ==
  data: u input; y output
function y = fcn(u)

% exponential scaling to enhance controls feeling:
e = 1.5; % [1:2]
y = [            u(1)   ;
      sign(u(2))*abs(u(2))^e ; 
      sign(u(3))*abs(u(3))^e ;
      sign(u(4))*abs(u(4))^e ];

== matlab function helicopter_sim/HELICOPTER MODEL/HELICOPTER FORCES AND MOMENTS/MAIN ROTOR/Stop simulation if retreating blade stalls /MATLAB Function ==
  data: u input
function fcn(u)

if u
    stall_mr = true;
    assignin('base', 'stall_mr', stall_mr);
else
    stall_mr = false;
    assignin('base', 'stall_mr', stall_mr);
end

== matlab function helicopter_sim/HELICOPTER MODEL/HELICOPTER FORCES AND MOMENTS/MAIN ROTOR/Stop simulation if retreating blade stalls /MATLAB Function1 ==
  data: alpha_loc input; alpha_max output
function alpha_max = fcn(alpha_loc)

alpha_max = max(alpha_loc(:));

== matlab function helicopter_sim/HELICOPTER MODEL/HELICOPTER FORCES AND MOMENTS/MAIN ROTOR/FLAPPING DYNAMICS (TIP-PATH-PLANE APPROX)/DAMPING MATRIX ==
  data: OMEGA input; GAMMA input; D output; EPSLN input; Mu input
function D = fcn(OMEGA,GAMMA,EPSLN,Mu)


D = OMEGA*[ 0.5*GAMMA*(1/4-2/3*EPSLN+0.5*EPSLN^2)                       0                      -GAMMA*Mu*1/4*(1/3-EPSLN+EPSLN^2)    ;
                           0                         0.5*GAMMA*(1/4-2/3*EPSLN+0.5*EPSLN^2)                      2                   ;
             -0.5*GAMMA*Mu*(1/3-EPSLN+EPSLN^2)                         -2                     0.5*GAMMA*(1/4-2/3*EPSLN+0.5*EPSLN^2) ];

== matlab function helicopter_sim/HELICOPTER MODEL/HELICOPTER FORCES AND MOMENTS/MAIN ROTOR/FLAPPING DYNAMICS (TIP-PATH-PLANE APPROX)/FORCING FUNCTION ==
  data: OMEGA input; GAMMA input; ROTOR input; f output; EPSLN input; Mu input; m_blade input; Jbeta input; Theta0 input; THETT input; A1s input; B1s input; lambda input; lambda_i input; pW input; qW input; pWdot input; qWdot input; beta_w input; g input
function f = fcn(OMEGA,GAMMA,ROTOR,EPSLN,Mu,m_blade,Jbeta,Theta0,THETT,A1s,B1s,lambda,lambda_i,pW,qW,pWdot,qWdot,beta_w,g)

Mbeta = g*1/2*m_blade*ROTOR^2*(1-EPSLN)^2; % weight moment of the blade around flap hinge (small flapping angle beta and level attitude) 
                                         % (distance from blade c.g. to flap hinge)*(blade weight) [N*m]
                                         % small contribution to the coning angle, can be neglected
% rotation of feathering angles from hub-body to hub-wind frame:
A1c = A1s*cos(beta_w)-B1s*sin(beta_w);
B1c = A1s*sin(beta_w)+B1s*cos(beta_w);
% calculation of the induced velocity coefficient K_iv for the triangular inflow model from Glauert:
% this models the slight contribution to lateral flapping of the higher inflow distribution on the aft part 
% of the rotor due to the wake being convected downstream in forward flight (see Leishman)
K_iv = 4/3*(Mu/lambda)/(1.2+Mu/lambda);


f1 = [ GAMMA/2*((1/4-EPSLN/3)+0.5*Mu^2*(1/2-EPSLN+0.5*EPSLN^2))    GAMMA/2*((1/5-EPSLN/4)+0.5*Mu^2*(1/3-EPSLN/2))                              0                                          -GAMMA*Mu/2*(1/3-EPSLN/2)                ;
                                      0                                                 0                           GAMMA/2*((1/4-EPSLN/3)+1/4*Mu^2*(1/2-EPSLN+0.5*EPSLN^2))                            0                          ;
                           -GAMMA*Mu/2*(2/3-EPSLN)                        -GAMMA*Mu/2*(1/2-2/3*EPSLN)                                          0                          GAMMA/2*((1/4-EPSLN/3)+3/4*Mu^2*(1/2-EPSLN+0.5*EPSLN^2)) ];

f2 = [    GAMMA*Mu/(8*OMEGA)*(2/3-EPSLN)                       0                              0           0           ;
       -2/OMEGA*(1+ROTOR*EPSLN*Mbeta/(g*Jbeta))     -GAMMA/(2*OMEGA)*(1/4-EPSLN/3)            0      -1/(OMEGA^2)     ;
          -GAMMA/(2*OMEGA)*(1/4-EPSLN/3)     2/OMEGA*(1+ROTOR*EPSLN*Mbeta/(g*Jbeta))    -1/(OMEGA^2)      0           ];

f3 = [         GAMMA/2*(1/3-EPSLN/2)                     0                ;
                         0                    GAMMA/2*K_iv*(1/4-EPSLN/3)  ;
       -GAMMA*Mu/2*(1/2-EPSLN+0.5*EPSLN^2)               0                ];

f4 = [ Mbeta/(g*Jbeta)*(-g) ;
               0            ;
               0            ];

f = OMEGA^2*(f1*[ Theta0 THETT A1c B1c ]') + ...
    OMEGA^2*(f2*[ pW qW pWdot qWdot ]')    + ...
    OMEGA^2*(f3*[ lambda -lambda_i ]') + f4;

== matlab function helicopter_sim/HELICOPTER MODEL/HELICOPTER FORCES AND MOMENTS/MAIN ROTOR/FLAPPING DYNAMICS (TIP-PATH-PLANE APPROX)/STIFFNESS MATRIX ==
  data: ROTOR input; OMEGA input; GAMMA input; K output; EPSLN input; Mu input; AKONE input; AKBETA input; m_blade input; Jbeta input; g input
function K = fcn(ROTOR,OMEGA,GAMMA,EPSLN,Mu,AKONE,AKBETA,m_blade,Jbeta,g)

Mbeta = g*1/2*m_blade*ROTOR^2*(1-EPSLN)^2; % weight moment of the blade around flap hinge (small flapping angle beta and level attitude) 
                                           % (distance from blade c.g. to flap hinge)*(blade weight) [N*m]
                                           % small contribution to the coning angle, can be neglected

P2 = 1 + AKBETA/(Jbeta*OMEGA^2) + EPSLN*ROTOR*Mbeta/(Jbeta*g) + GAMMA*AKONE/8*(1-4/3*EPSLN); % squared ratio of flapping frequency and rotor angular speed

K = OMEGA^2*[ P2+GAMMA*AKONE*Mu^2*1/4*(1/2-EPSLN+0.5*EPSLN^2)            -GAMMA*Mu*1/4*(0.5*EPSLN-EPSLN^2)                                     -GAMMA*AKONE*Mu*1/4*(2/3-EPSLN)                              ;
                       -GAMMA*Mu*1/2*(1/3-0.5*EPSLN)                P2-1+GAMMA*AKONE*Mu^2*1/8*(1/2-EPSLN+0.5*EPSLN^2)          0.5*GAMMA*(1/4-2/3*EPSLN+0.5*EPSLN^2)+GAMMA*Mu^2*1/8*(1/2-EPSLN+0.5*EPSLN^2) ;
                      -GAMMA*AKONE*Mu*0.5*(2/3-EPSLN)   -0.5*GAMMA*(1/4-2/3*EPSLN+0.5*EPSLN^2)+GAMMA*Mu^2*1/8*(1/2-EPSLN+0.5*EPSLN^2)   P2-1+GAMMA*AKONE*Mu^2*3/8*(1/2-EPSLN+0.5*EPSLN^2)                   ];

== matlab function helicopter_sim/HELICOPTER MODEL/HELICOPTER FORCES AND MOMENTS/MAIN ROTOR/FLAPPING DYNAMICS (TIP-PATH-PLANE APPROX)/calculate sidesplip ==
  data: Mu output; chi input; beta_w output; i_s input; OMEGA input; ROTOR input; STACG input; BLCG input; WLCG input; STAH input; BLH input; WLH input; TAS input; omega_TAS input
function [Mu,beta_w] = fcn(chi,i_s,OMEGA,ROTOR,STACG,BLCG,WLCG,STAH,BLH,WLH,TAS,omega_TAS)

% calculate sideslip:
lever_arm_H = [STACG-STAH BLH-BLCG WLCG-WLH]'; % vector from cg to rotor hub
TAS_H = [1 chi 1]'.*(TAS + cross(omega_TAS,lever_arm_H)); % wind speed at rotor
% rotation of airspeed from body to hub-body frame:
uH = TAS_H(1)*cos(i_s)-TAS_H(3)*sin(i_s);
vH = TAS_H(2);
wH = TAS_H(1)*sin(i_s)+TAS_H(3)*cos(i_s);
beta_w = atan2(vH,uH); % sideslip angle 
Mu = sqrt(uH^2+vH^2)/(OMEGA*ROTOR); % advance ratio

== matlab function helicopter_sim/HELICOPTER MODEL/HELICOPTER FORCES AND MOMENTS/MAIN ROTOR/FLAPPING DYNAMICS (TIP-PATH-PLANE APPROX)/flapping restraint ==
  data: max_flap input; a output; a input; stop output
function [a,stop] = fcn(max_flap,a)

a0 = a(1); a1 = a(2); b1 = a(3);

beta_max = a0 + sqrt(a1^2+b1^2);
beta_min = a0 - sqrt(a1^2+b1^2);

flag = false;
if abs(beta_max)>max_flap ||  abs(beta_min)>max_flap
    
    %k = max_flap/(abs(a0)+sqrt(a1^2+b1^2)); %scaling factor
    k = sqrt((max_flap-abs(a0))^2)/sqrt(a1^2+b1^2); %scaling factor (coning unaltered)
    %a = k*[ a0 a1 b1 ]';
    a = [ a0 k*a1 k*b1 ]';
    flag = true;
    stop = true;
else
    a = [ a0 a1 b1 ]';
    stop = false;
end

if flag
    over_flap = true;
    assignin('base', 'over_flap', over_flap);
else
    over_flap = false;
    assignin('base', 'over_flap', over_flap);
end

== matlab function helicopter_sim/HELICOPTER MODEL/HELICOPTER FORCES AND MOMENTS/MAIN ROTOR/FLAPPING DYNAMICS (TIP-PATH-PLANE APPROX)/hub-wind axis rotation of angular rates ==
  data: chi input; omega input; omegadot input; pW output; qW output; pWdot output; qWdot output; i_s input; beta_w input
function [pW,qW,pWdot,qWdot] = fcn(chi,omega,omegadot,i_s,beta_w)

p = omega(1); % roll rate
q = omega(2); % pitch rate
r = omega(3); % yaw rate
pH = chi*(p*cos(i_s)+r*sin(i_s));
qH = q;
pdot = omegadot(1); % roll acceleration 
qdot = omegadot(2); % pitch acceleration 
rdot = omegadot(3); % yaw acceleration 
pHdot = chi*(pdot*cos(i_s)+rdot*sin(i_s));
qHdot = qdot;
pW = pH*cos(beta_w)+qH*sin(beta_w);
qW = -pH*sin(beta_w)+qH*cos(beta_w);
pWdot = pHdot*cos(beta_w)+qHdot*sin(beta_w);
qWdot = -pHdot*sin(beta_w)+qHdot*cos(beta_w);

== matlab function helicopter_sim/HELICOPTER MODEL/HELICOPTER FORCES AND MOMENTS/MAIN ROTOR/FLAPPING DYNAMICS (TIP-PATH-PLANE APPROX)/rotation from hub-body to hub-wind ==
  data: a_b input; beta_w input; a_w output
function a_w = fcn(a_b,beta_w)

% rotate flapping angles:
a1s = a_b(2); b1s = a_b(3);
a1w = a1s*cos(beta_w)-b1s*sin(beta_w);
b1w = a1s*sin(beta_w)+b1s*cos(beta_w);

a_w = [a_b(1);a1w;b1w];

== matlab function helicopter_sim/HELICOPTER MODEL/HELICOPTER FORCES AND MOMENTS/MAIN ROTOR/FLAPPING DYNAMICS (TIP-PATH-PLANE APPROX)/rotation from hub-wind to hub-body ==
  data: a input; beta_w input; a1s output; b1s output
function [a1s,b1s] = fcn(a,beta_w)

a1 = a(2); b1 = a(3);

a1s = a1*cos(beta_w)+b1*sin(beta_w);
b1s = -a1*sin(beta_w)+b1*cos(beta_w);

== matlab function helicopter_sim/HELICOPTER MODEL/HELICOPTER FORCES AND MOMENTS/FUSELAGE /FUSELAGE AERODYNAMIC FORCES ==
  data: lambda_i input; CL_f input; CD_f input; CY_f input; CLL_f input; CM_f input; CN_f input; STARPF input; BLRPF input; WLRPF input; STACG input; BLCG input; WLCG input; rho input; TAS input; F_fuselage output; M_fuselage output; OMEGA input; ROTOR input
function [F_fuselage, M_fuselage] = fcn(lambda_i,CL_f,CD_f,CY_f,CLL_f,CM_f,CN_f,STARPF,BLRPF,WLRPF,STACG,BLCG,WLCG,rho,TAS,OMEGA,ROTOR)

%% preliminary calculations
% rotor downwash on fuselage:
% simply the value of induced velocity at the rotor disk (fuselage is considered to be placed in the very near wake)
% reminder: induced velocity ratio is positive when going up through the main rotor
w_if = (lambda_i)*OMEGA*ROTOR;
% fuselage angle of attack and of sideslip calculation in body axis:
u_f = TAS(1);
v_f = TAS(2);
w_f = TAS(3);
V_f = sqrt(u_f^2+v_f^2+w_f^2);
alpha_f = atan2(w_f+w_if,u_f);
if V_f == 0
    beta_f = 0;
else
    beta_f = asin(v_f/V_f);
end
q_f     = 0.5*rho*V_f^2;

%% aerodynamic forces
L_f  = (CL_f(1)+CL_f(2)*alpha_f)*q_f; % lift
Y_f  = (CY_f(1)+CY_f(2)*beta_f)*q_f; % sideforce
D_f  = (CD_f(1)+CD_f(2)*alpha_f+CD_f(3)*alpha_f^2)*q_f; % drag
LL_f = (CLL_f(1)+CLL_f(2)*beta_f)*q_f; % rolling moment
M_f  = (CM_f(1)+CM_f(2)*alpha_f)*q_f; % pitching moment
N_f  = (CN_f(1)+CN_f(2)*beta_f)*q_f; % yawing moment 

%% forces and moments acting on cg in body axis
lever_arm_cp = [STACG-STARPF BLRPF-BLCG WLCG-WLRPF]';
X  = -D_f*cos(beta_f)*cos(alpha_f)-Y_f*sin(beta_f)*sin(alpha_f)+L_f*sin(alpha_f);
Y  = Y_f*cos(beta_f)-D_f*sin(beta_f);
Z  = -L_f*cos(alpha_f)-D_f*cos(beta_f)*sin(alpha_f)-Y_f*sin(beta_f)*sin(alpha_f);
LL = LL_f*cos(beta_f)*cos(alpha_f)-M_f*sin(beta_f)*cos(alpha_f)-N_f*sin(alpha_f);
M  = M_f*cos(beta_f)+LL_f*sin(beta_f);
N  = N_f*cos(alpha_f)+LL_f*cos(beta_f)*cos(alpha_f)-M_f*sin(beta_f)*sin(alpha_f);
F_fuselage = [ X Y Z ]';
M_fuselage = [ LL M N ]' + cross(lever_arm_cp,F_fuselage);

% neglect contribution near hover:
if abs(V_f)<1
    F_fuselage = [ 0 0 0 ]';
    M_fuselage = [ 0 0 0 ]';
end

% %% simplified equivalent flat plate drag area model 
% lever_arm_cp = [STACG-STARPF BLRPF-BLCG WLCG-WLRPF]';
% f = 19.3*0.3048^2; %fuselage parasite drag area [ft^2-->m^2]
% Ax = f; Ay = f*1.5; Az = f*1.5;
% F_fuselage = -0.5*rho*[TAS(1)*Ax TAS(2)*Ay TAS(3)*Az]'*norm(TAS);
% M_fuselage = cross(lever_arm_cp,F_fuselage);
